simulink model "TSR_Scenario_002_cs"  (R2014b)
(part 2 of 39)

      mask help:
      | The VisuMatrixSign block provides a way to adapt the texture of the plates connected to an overhang, based on Resource IDs of the texture files.
      |
      | For more information, please click Help.
      settings: OpenFcn=open_system([gcb '/Actuator'],'mask')
      mask Help: eval('openHelp(733)')
      mask Display: image(imread('HighwaySpeedMatrix.png'))
  VISUMatrixSign_HighwayOverhang_21 : Subsystem  Tag=actuator/VisuMatrixSign  Priority=0  mask(PreScan Sink Block: VisuMatrixSign){UniqueID=1099, ResourceList={'1' 'InformationSign\MatrixSign_GreenArrow.png' '2' 'InformationSign\Empty.jpeg' '3' 'InformationSign\SEARCH_Logo.png' '4' 'InformationSign\z274-50_black_full.png' '5' 'InformationSign\z274-51_black_full.png' '6' 'InformationSign\z274-52_black_full.png' '7' 'InformationSign\z274-53_black_full.png' '8' 'InformationSign\z274-54_black_full.png' '9' 'InformationSign\z274-55_black_full.png' '10' 'InformationSign\z274-56_black_full.png' '11' 'InformationSign\z274-57_black_full.png' '12' 'InformationSign\z274-58_black_full.png' '13' 'InformationSign\z274-59_black_full.png' '14' 'InformationSign\z274-60_black_full.png' '15' 'InformationSign\z274-61_black_full.png' '16' 'InformationSign\z274-62_black_full.png' '17' 'InformationSign\z274-63_black_full.png' }, PivotName=}
      mask prompts: UniqueID "Parent Unique Identifier (auto-generated)"; ResourceList "Resource List (auto-generated)"; PivotName "Name of pivot (auto-generated)"
      mask help:
      | The VisuMatrixSign block provides a way to adapt the texture of the plates connected to an overhang, based on Resource IDs of the texture files.
      |
      | For more information, please click Help.
      settings: OpenFcn=open_system([gcb '/Actuator'],'mask')
      mask Help: eval('openHelp(733)')
      mask Display: image(imread('HighwaySpeedMatrix.png'))
  VISUMatrixSign_HighwayOverhang_22 : Subsystem  Tag=actuator/VisuMatrixSign  Priority=0  mask(PreScan Sink Block: VisuMatrixSign){UniqueID=1100, ResourceList={'1' 'InformationSign\MatrixSign_GreenArrow.png' '2' 'InformationSign\Empty.jpeg' '3' 'InformationSign\SEARCH_Logo.png' '4' 'InformationSign\z274-50_black_full.png' '5' 'InformationSign\z274-51_black_full.png' '6' 'InformationSign\z274-52_black_full.png' '7' 'InformationSign\z274-53_black_full.png' '8' 'InformationSign\z274-54_black_full.png' '9' 'InformationSign\z274-55_black_full.png' '10' 'InformationSign\z274-56_black_full.png' '11' 'InformationSign\z274-57_black_full.png' '12' 'InformationSign\z274-58_black_full.png' '13' 'InformationSign\z274-59_black_full.png' '14' 'InformationSign\z274-60_black_full.png' '15' 'InformationSign\z274-61_black_full.png' '16' 'InformationSign\z274-62_black_full.png' '17' 'InformationSign\z274-63_black_full.png' }, PivotName=}
      mask prompts: UniqueID "Parent Unique Identifier (auto-generated)"; ResourceList "Resource List (auto-generated)"; PivotName "Name of pivot (auto-generated)"
      mask help:
      | The VisuMatrixSign block provides a way to adapt the texture of the plates connected to an overhang, based on Resource IDs of the texture files.
      |
      | For more information, please click Help.
      settings: OpenFcn=open_system([gcb '/Actuator'],'mask')
      mask Help: eval('openHelp(733)')
      mask Display: image(imread('HighwaySpeedMatrix.png'))
  VISUMatrixSign_HighwayOverhang_23 : Subsystem  Tag=actuator/VisuMatrixSign  Priority=0  mask(PreScan Sink Block: VisuMatrixSign){UniqueID=1102, ResourceList={'1' 'InformationSign\MatrixSign_GreenArrow.png' '2' 'InformationSign\Empty.jpeg' '3' 'InformationSign\SEARCH_Logo.png' '4' 'InformationSign\z274-50_black_full.png' '5' 'InformationSign\z274-51_black_full.png' '6' 'InformationSign\z274-52_black_full.png' '7' 'InformationSign\z274-53_black_full.png' '8' 'InformationSign\z274-54_black_full.png' '9' 'InformationSign\z274-55_black_full.png' '10' 'InformationSign\z274-56_black_full.png' '11' 'InformationSign\z274-57_black_full.png' '12' 'InformationSign\z274-58_black_full.png' '13' 'InformationSign\z274-59_black_full.png' '14' 'InformationSign\z274-60_black_full.png' '15' 'InformationSign\z274-61_black_full.png' '16' 'InformationSign\z274-62_black_full.png' '17' 'InformationSign\z274-63_black_full.png' }, PivotName=}
      mask prompts: UniqueID "Parent Unique Identifier (auto-generated)"; ResourceList "Resource List (auto-generated)"; PivotName "Name of pivot (auto-generated)"
      mask help:
      | The VisuMatrixSign block provides a way to adapt the texture of the plates connected to an overhang, based on Resource IDs of the texture files.
      |
      | For more information, please click Help.
      settings: OpenFcn=open_system([gcb '/Actuator'],'mask')
      mask Help: eval('openHelp(733)')
      mask Display: image(imread('HighwaySpeedMatrix.png'))
  VISUMatrixSign_HighwayOverhang_24 : Subsystem  Tag=actuator/VisuMatrixSign  Priority=0  mask(PreScan Sink Block: VisuMatrixSign){UniqueID=1103, ResourceList={'1' 'InformationSign\MatrixSign_GreenArrow.png' '2' 'InformationSign\Empty.jpeg' '3' 'InformationSign\SEARCH_Logo.png' '4' 'InformationSign\z274-50_black_full.png' '5' 'InformationSign\z274-51_black_full.png' '6' 'InformationSign\z274-52_black_full.png' '7' 'InformationSign\z274-53_black_full.png' '8' 'InformationSign\z274-54_black_full.png' '9' 'InformationSign\z274-55_black_full.png' '10' 'InformationSign\z274-56_black_full.png' '11' 'InformationSign\z274-57_black_full.png' '12' 'InformationSign\z274-58_black_full.png' '13' 'InformationSign\z274-59_black_full.png' '14' 'InformationSign\z274-60_black_full.png' '15' 'InformationSign\z274-61_black_full.png' '16' 'InformationSign\z274-62_black_full.png' '17' 'InformationSign\z274-63_black_full.png' }, PivotName=}
      mask prompts: UniqueID "Parent Unique Identifier (auto-generated)"; ResourceList "Resource List (auto-generated)"; PivotName "Name of pivot (auto-generated)"
      mask help:
      | The VisuMatrixSign block provides a way to adapt the texture of the plates connected to an overhang, based on Resource IDs of the texture files.
      |
      | For more information, please click Help.
      settings: OpenFcn=open_system([gcb '/Actuator'],'mask')
      mask Help: eval('openHelp(733)')
      mask Display: image(imread('HighwaySpeedMatrix.png'))
  VISUMatrixSign_HighwayOverhang_25 : Subsystem  Tag=actuator/VisuMatrixSign  Priority=0  mask(PreScan Sink Block: VisuMatrixSign){UniqueID=1104, ResourceList={'1' 'InformationSign\MatrixSign_GreenArrow.png' '2' 'InformationSign\Empty.jpeg' '3' 'InformationSign\SEARCH_Logo.png' '4' 'InformationSign\z274-50_black_full.png' '5' 'InformationSign\z274-51_black_full.png' '6' 'InformationSign\z274-52_black_full.png' '7' 'InformationSign\z274-53_black_full.png' '8' 'InformationSign\z274-54_black_full.png' '9' 'InformationSign\z274-55_black_full.png' '10' 'InformationSign\z274-56_black_full.png' '11' 'InformationSign\z274-57_black_full.png' '12' 'InformationSign\z274-58_black_full.png' '13' 'InformationSign\z274-59_black_full.png' '14' 'InformationSign\z274-60_black_full.png' '15' 'InformationSign\z274-61_black_full.png' '16' 'InformationSign\z274-62_black_full.png' '17' 'InformationSign\z274-63_black_full.png' }, PivotName=}
      mask prompts: UniqueID "Parent Unique Identifier (auto-generated)"; ResourceList "Resource List (auto-generated)"; PivotName "Name of pivot (auto-generated)"
      mask help:
      | The VisuMatrixSign block provides a way to adapt the texture of the plates connected to an overhang, based on Resource IDs of the texture files.
      |
      | For more information, please click Help.
      settings: OpenFcn=open_system([gcb '/Actuator'],'mask')
      mask Help: eval('openHelp(733)')
      mask Display: image(imread('HighwaySpeedMatrix.png'))
  VISUMatrixSign_HighwayOverhang_26 : Subsystem  Tag=actuator/VisuMatrixSign  Priority=0  mask(PreScan Sink Block: VisuMatrixSign){UniqueID=1105, ResourceList={'1' 'InformationSign\MatrixSign_GreenArrow.png' '2' 'InformationSign\Empty.jpeg' '3' 'InformationSign\SEARCH_Logo.png' '4' 'InformationSign\z274-50_black_full.png' '5' 'InformationSign\z274-51_black_full.png' '6' 'InformationSign\z274-52_black_full.png' '7' 'InformationSign\z274-53_black_full.png' '8' 'InformationSign\z274-54_black_full.png' '9' 'InformationSign\z274-55_black_full.png' '10' 'InformationSign\z274-56_black_full.png' '11' 'InformationSign\z274-57_black_full.png' '12' 'InformationSign\z274-58_black_full.png' '13' 'InformationSign\z274-59_black_full.png' '14' 'InformationSign\z274-60_black_full.png' '15' 'InformationSign\z274-61_black_full.png' '16' 'InformationSign\z274-62_black_full.png' '17' 'InformationSign\z274-63_black_full.png' }, PivotName=}
      mask prompts: UniqueID "Parent Unique Identifier (auto-generated)"; ResourceList "Resource List (auto-generated)"; PivotName "Name of pivot (auto-generated)"
      mask help:
      | The VisuMatrixSign block provides a way to adapt the texture of the plates connected to an overhang, based on Resource IDs of the texture files.
      |
      | For more information, please click Help.
      settings: OpenFcn=open_system([gcb '/Actuator'],'mask')
      mask Help: eval('openHelp(733)')
      mask Display: image(imread('HighwaySpeedMatrix.png'))
  VISUMatrixSign_HighwayOverhang_27 : Subsystem  Tag=actuator/VisuMatrixSign  Priority=0  mask(PreScan Sink Block: VisuMatrixSign){UniqueID=1106, ResourceList={'1' 'InformationSign\MatrixSign_GreenArrow.png' '2' 'InformationSign\Empty.jpeg' '3' 'InformationSign\SEARCH_Logo.png' '4' 'InformationSign\z274-50_black_full.png' '5' 'InformationSign\z274-51_black_full.png' '6' 'InformationSign\z274-52_black_full.png' '7' 'InformationSign\z274-53_black_full.png' '8' 'InformationSign\z274-54_black_full.png' '9' 'InformationSign\z274-55_black_full.png' '10' 'InformationSign\z274-56_black_full.png' '11' 'InformationSign\z274-57_black_full.png' '12' 'InformationSign\z274-58_black_full.png' '13' 'InformationSign\z274-59_black_full.png' '14' 'InformationSign\z274-60_black_full.png' '15' 'InformationSign\z274-61_black_full.png' '16' 'InformationSign\z274-62_black_full.png' '17' 'InformationSign\z274-63_black_full.png' }, PivotName=}
      mask prompts: UniqueID "Parent Unique Identifier (auto-generated)"; ResourceList "Resource List (auto-generated)"; PivotName "Name of pivot (auto-generated)"
      mask help:
      | The VisuMatrixSign block provides a way to adapt the texture of the plates connected to an overhang, based on Resource IDs of the texture files.
      |
      | For more information, please click Help.
      settings: OpenFcn=open_system([gcb '/Actuator'],'mask')
      mask Help: eval('openHelp(733)')
      mask Display: image(imread('HighwaySpeedMatrix.png'))
  VISUMatrixSign_HighwayOverhang_28 : Subsystem  Tag=actuator/VisuMatrixSign  Priority=0  mask(PreScan Sink Block: VisuMatrixSign){UniqueID=1107, ResourceList={'1' 'InformationSign\MatrixSign_GreenArrow.png' '2' 'InformationSign\Empty.jpeg' '3' 'InformationSign\SEARCH_Logo.png' '4' 'InformationSign\z274-50_black_full.png' '5' 'InformationSign\z274-51_black_full.png' '6' 'InformationSign\z274-52_black_full.png' '7' 'InformationSign\z274-53_black_full.png' '8' 'InformationSign\z274-54_black_full.png' '9' 'InformationSign\z274-55_black_full.png' '10' 'InformationSign\z274-56_black_full.png' '11' 'InformationSign\z274-57_black_full.png' '12' 'InformationSign\z274-58_black_full.png' '13' 'InformationSign\z274-59_black_full.png' '14' 'InformationSign\z274-60_black_full.png' '15' 'InformationSign\z274-61_black_full.png' '16' 'InformationSign\z274-62_black_full.png' '17' 'InformationSign\z274-63_black_full.png' }, PivotName=}
      mask prompts: UniqueID "Parent Unique Identifier (auto-generated)"; ResourceList "Resource List (auto-generated)"; PivotName "Name of pivot (auto-generated)"
      mask help:
      | The VisuMatrixSign block provides a way to adapt the texture of the plates connected to an overhang, based on Resource IDs of the texture files.
      |
      | For more information, please click Help.
      settings: OpenFcn=open_system([gcb '/Actuator'],'mask')
      mask Help: eval('openHelp(733)')
      mask Display: image(imread('HighwaySpeedMatrix.png'))
  VISUMatrixSign_HighwayOverhang_3 : Subsystem  Tag=actuator/VisuMatrixSign  Priority=0  mask(PreScan Sink Block: VisuMatrixSign){UniqueID=440, ResourceList={'1' 'InformationSign\MatrixSign_GreenArrow.png' '2' 'InformationSign\Empty.jpeg' '3' 'InformationSign\SEARCH_Logo.png' '4' 'InformationSign\z274-50_black_full.png' '5' 'InformationSign\z274-51_black_full.png' '6' 'InformationSign\z274-52_black_full.png' '7' 'InformationSign\z274-53_black_full.png' '8' 'InformationSign\z274-54_black_full.png' '9' 'InformationSign\z274-55_black_full.png' '10' 'InformationSign\z274-56_black_full.png' '11' 'InformationSign\z274-57_black_full.png' '12' 'InformationSign\z274-58_black_full.png' '13' 'InformationSign\z274-59_black_full.png' '14' 'InformationSign\z274-60_black_full.png' '15' 'InformationSign\z274-61_black_full.png' '16' 'InformationSign\z274-62_black_full.png' '17' 'InformationSign\z274-63_black_full.png' }, PivotName=}
      mask prompts: UniqueID "Parent Unique Identifier (auto-generated)"; ResourceList "Resource List (auto-generated)"; PivotName "Name of pivot (auto-generated)"
      mask help:
      | The VisuMatrixSign block provides a way to adapt the texture of the plates connected to an overhang, based on Resource IDs of the texture files.
      |
      | For more information, please click Help.
      settings: OpenFcn=open_system([gcb '/Actuator'],'mask')
      mask Help: eval('openHelp(733)')
      mask Display: image(imread('HighwaySpeedMatrix.png'))
  VISUMatrixSign_HighwayOverhang_4 : Subsystem  Tag=actuator/VisuMatrixSign  Priority=0  mask(PreScan Sink Block: VisuMatrixSign){UniqueID=441, ResourceList={'1' 'InformationSign\MatrixSign_GreenArrow.png' '2' 'InformationSign\Empty.jpeg' '3' 'InformationSign\SEARCH_Logo.png' '4' 'InformationSign\z274-50_black_full.png' '5' 'InformationSign\z274-51_black_full.png' '6' 'InformationSign\z274-52_black_full.png' '7' 'InformationSign\z274-53_black_full.png' '8' 'InformationSign\z274-54_black_full.png' '9' 'InformationSign\z274-55_black_full.png' '10' 'InformationSign\z274-56_black_full.png' '11' 'InformationSign\z274-57_black_full.png' '12' 'InformationSign\z274-58_black_full.png' '13' 'InformationSign\z274-59_black_full.png' '14' 'InformationSign\z274-60_black_full.png' '15' 'InformationSign\z274-61_black_full.png' '16' 'InformationSign\z274-62_black_full.png' '17' 'InformationSign\z274-63_black_full.png' }, PivotName=}
      mask prompts: UniqueID "Parent Unique Identifier (auto-generated)"; ResourceList "Resource List (auto-generated)"; PivotName "Name of pivot (auto-generated)"
      mask help:
      | The VisuMatrixSign block provides a way to adapt the texture of the plates connected to an overhang, based on Resource IDs of the texture files.
      |
      | For more information, please click Help.
      settings: OpenFcn=open_system([gcb '/Actuator'],'mask')
      mask Help: eval('openHelp(733)')
      mask Display: image(imread('HighwaySpeedMatrix.png'))
  VISUMatrixSign_HighwayOverhang_5 : Subsystem  Tag=actuator/VisuMatrixSign  Priority=0  mask(PreScan Sink Block: VisuMatrixSign){UniqueID=843, ResourceList={'1' 'InformationSign\MatrixSign_GreenArrow.png' '2' 'InformationSign\Empty.jpeg' '3' 'InformationSign\SEARCH_Logo.png' '4' 'InformationSign\z274-50_black_full.png' '5' 'InformationSign\z274-51_black_full.png' '6' 'InformationSign\z274-52_black_full.png' '7' 'InformationSign\z274-53_black_full.png' '8' 'InformationSign\z274-54_black_full.png' '9' 'InformationSign\z274-55_black_full.png' '10' 'InformationSign\z274-56_black_full.png' '11' 'InformationSign\z274-57_black_full.png' '12' 'InformationSign\z274-58_black_full.png' '13' 'InformationSign\z274-59_black_full.png' '14' 'InformationSign\z274-60_black_full.png' '15' 'InformationSign\z274-61_black_full.png' '16' 'InformationSign\z274-62_black_full.png' '17' 'InformationSign\z274-63_black_full.png' }, PivotName=}
      mask prompts: UniqueID "Parent Unique Identifier (auto-generated)"; ResourceList "Resource List (auto-generated)"; PivotName "Name of pivot (auto-generated)"
      mask help:
      | The VisuMatrixSign block provides a way to adapt the texture of the plates connected to an overhang, based on Resource IDs of the texture files.
      |
      | For more information, please click Help.
      settings: OpenFcn=open_system([gcb '/Actuator'],'mask')
      mask Help: eval('openHelp(733)')
      mask Display: image(imread('HighwaySpeedMatrix.png'))
  VISUMatrixSign_HighwayOverhang_6 : Subsystem  Tag=actuator/VisuMatrixSign  Priority=0  mask(PreScan Sink Block: VisuMatrixSign){UniqueID=846, ResourceList={'1' 'InformationSign\MatrixSign_GreenArrow.png' '2' 'InformationSign\Empty.jpeg' '3' 'InformationSign\SEARCH_Logo.png' '4' 'InformationSign\z274-50_black_full.png' '5' 'InformationSign\z274-51_black_full.png' '6' 'InformationSign\z274-52_black_full.png' '7' 'InformationSign\z274-53_black_full.png' '8' 'InformationSign\z274-54_black_full.png' '9' 'InformationSign\z274-55_black_full.png' '10' 'InformationSign\z274-56_black_full.png' '11' 'InformationSign\z274-57_black_full.png' '12' 'InformationSign\z274-58_black_full.png' '13' 'InformationSign\z274-59_black_full.png' '14' 'InformationSign\z274-60_black_full.png' '15' 'InformationSign\z274-61_black_full.png' '16' 'InformationSign\z274-62_black_full.png' '17' 'InformationSign\z274-63_black_full.png' }, PivotName=}
      mask prompts: UniqueID "Parent Unique Identifier (auto-generated)"; ResourceList "Resource List (auto-generated)"; PivotName "Name of pivot (auto-generated)"
      mask help:
      | The VisuMatrixSign block provides a way to adapt the texture of the plates connected to an overhang, based on Resource IDs of the texture files.
      |
      | For more information, please click Help.
      settings: OpenFcn=open_system([gcb '/Actuator'],'mask')
      mask Help: eval('openHelp(733)')
      mask Display: image(imread('HighwaySpeedMatrix.png'))
  VISUMatrixSign_HighwayOverhang_7 : Subsystem  Tag=actuator/VisuMatrixSign  Priority=0  mask(PreScan Sink Block: VisuMatrixSign){UniqueID=867, ResourceList={'1' 'InformationSign\MatrixSign_GreenArrow.png' '2' 'InformationSign\Empty.jpeg' '3' 'InformationSign\SEARCH_Logo.png' '4' 'InformationSign\z274-50_black_full.png' '5' 'InformationSign\z274-51_black_full.png' '6' 'InformationSign\z274-52_black_full.png' '7' 'InformationSign\z274-53_black_full.png' '8' 'InformationSign\z274-54_black_full.png' '9' 'InformationSign\z274-55_black_full.png' '10' 'InformationSign\z274-56_black_full.png' '11' 'InformationSign\z274-57_black_full.png' '12' 'InformationSign\z274-58_black_full.png' '13' 'InformationSign\z274-59_black_full.png' '14' 'InformationSign\z274-60_black_full.png' '15' 'InformationSign\z274-61_black_full.png' '16' 'InformationSign\z274-62_black_full.png' '17' 'InformationSign\z274-63_black_full.png' }, PivotName=}
      mask prompts: UniqueID "Parent Unique Identifier (auto-generated)"; ResourceList "Resource List (auto-generated)"; PivotName "Name of pivot (auto-generated)"
      mask help:
      | The VisuMatrixSign block provides a way to adapt the texture of the plates connected to an overhang, based on Resource IDs of the texture files.
      |
      | For more information, please click Help.
      settings: OpenFcn=open_system([gcb '/Actuator'],'mask')
      mask Help: eval('openHelp(733)')
      mask Display: image(imread('HighwaySpeedMatrix.png'))
  VISUMatrixSign_HighwayOverhang_8 : Subsystem  Tag=actuator/VisuMatrixSign  Priority=0  mask(PreScan Sink Block: VisuMatrixSign){UniqueID=870, ResourceList={'1' 'InformationSign\MatrixSign_GreenArrow.png' '2' 'InformationSign\Empty.jpeg' '3' 'InformationSign\SEARCH_Logo.png' '4' 'InformationSign\z274-50_black_full.png' '5' 'InformationSign\z274-51_black_full.png' '6' 'InformationSign\z274-52_black_full.png' '7' 'InformationSign\z274-53_black_full.png' '8' 'InformationSign\z274-54_black_full.png' '9' 'InformationSign\z274-55_black_full.png' '10' 'InformationSign\z274-56_black_full.png' '11' 'InformationSign\z274-57_black_full.png' '12' 'InformationSign\z274-58_black_full.png' '13' 'InformationSign\z274-59_black_full.png' '14' 'InformationSign\z274-60_black_full.png' '15' 'InformationSign\z274-61_black_full.png' '16' 'InformationSign\z274-62_black_full.png' '17' 'InformationSign\z274-63_black_full.png' }, PivotName=}
      mask prompts: UniqueID "Parent Unique Identifier (auto-generated)"; ResourceList "Resource List (auto-generated)"; PivotName "Name of pivot (auto-generated)"
      mask help:
      | The VisuMatrixSign block provides a way to adapt the texture of the plates connected to an overhang, based on Resource IDs of the texture files.
      |
      | For more information, please click Help.
      settings: OpenFcn=open_system([gcb '/Actuator'],'mask')
      mask Help: eval('openHelp(733)')
      mask Display: image(imread('HighwaySpeedMatrix.png'))
  VISUMatrixSign_HighwayOverhang_9 : Subsystem  Tag=actuator/VisuMatrixSign  Priority=0  mask(PreScan Sink Block: VisuMatrixSign){UniqueID=875, ResourceList={'1' 'InformationSign\MatrixSign_GreenArrow.png' '2' 'InformationSign\Empty.jpeg' '3' 'InformationSign\SEARCH_Logo.png' '4' 'InformationSign\z274-50_black_full.png' '5' 'InformationSign\z274-51_black_full.png' '6' 'InformationSign\z274-52_black_full.png' '7' 'InformationSign\z274-53_black_full.png' '8' 'InformationSign\z274-54_black_full.png' '9' 'InformationSign\z274-55_black_full.png' '10' 'InformationSign\z274-56_black_full.png' '11' 'InformationSign\z274-57_black_full.png' '12' 'InformationSign\z274-58_black_full.png' '13' 'InformationSign\z274-59_black_full.png' '14' 'InformationSign\z274-60_black_full.png' '15' 'InformationSign\z274-61_black_full.png' '16' 'InformationSign\z274-62_black_full.png' '17' 'InformationSign\z274-63_black_full.png' }, PivotName=}
      mask prompts: UniqueID "Parent Unique Identifier (auto-generated)"; ResourceList "Resource List (auto-generated)"; PivotName "Name of pivot (auto-generated)"
      mask help:
      | The VisuMatrixSign block provides a way to adapt the texture of the plates connected to an overhang, based on Resource IDs of the texture files.
      |
      | For more information, please click Help.
      settings: OpenFcn=open_system([gcb '/Actuator'],'mask')
      mask Help: eval('openHelp(733)')
      mask Display: image(imread('HighwaySpeedMatrix.png'))
  WheelL0_Audi_A8_1 : Subsystem  Tag=Actuator  Priority=0  LoadFcn=load('PrescanPoseData');load('PrescanXYZData');load('PreScanRPYData')
      mask help:
      | The VisuJoint block provides a way to adapt the location and orientation of a part of an object.
      |
      | For more information, please click Help.
      settings: OpenFcn=open_system([gcb '/Actuator'],'mask')
      mask Display: image(imread('Joint.png'))
  WheelL0_BMW_X5_2 : Subsystem  Tag=Actuator  Priority=0  LoadFcn=load('PrescanPoseData');load('PrescanXYZData');load('PreScanRPYData')
      mask help:
      | The VisuJoint block provides a way to adapt the location and orientation of a part of an object.
      |
      | For more information, please click Help.
      settings: OpenFcn=open_system([gcb '/Actuator'],'mask')
      mask Display: image(imread('Joint.png'))
  WheelL0_Citroen_C3_1 : Subsystem  Tag=Actuator  Priority=0  LoadFcn=load('PrescanPoseData');load('PrescanXYZData');load('PreScanRPYData')
      mask help:
      | The VisuJoint block provides a way to adapt the location and orientation of a part of an object.
      |
      | For more information, please click Help.
      settings: OpenFcn=open_system([gcb '/Actuator'],'mask')
      mask Display: image(imread('Joint.png'))
  WheelL0_Fiat_Bravo_1 : Subsystem  Tag=Actuator  Priority=0  LoadFcn=load('PrescanPoseData');load('PrescanXYZData');load('PreScanRPYData')
      mask help:
      | The VisuJoint block provides a way to adapt the location and orientation of a part of an object.
      |
      | For more information, please click Help.
      settings: OpenFcn=open_system([gcb '/Actuator'],'mask')
      mask Display: image(imread('Joint.png'))
  WheelL0_Nissan_Cabstar_1 : Subsystem  Tag=Actuator  Priority=0  LoadFcn=load('PrescanPoseData');load('PrescanXYZData');load('PreScanRPYData')
      mask help:
      | The VisuJoint block provides a way to adapt the location and orientation of a part of an object.
      |
      | For more information, please click Help.
      settings: OpenFcn=open_system([gcb '/Actuator'],'mask')
      mask Display: image(imread('Joint.png'))
  WheelL1_Audi_A8_1 : Subsystem  Tag=Actuator  Priority=0  LoadFcn=load('PrescanPoseData');load('PrescanXYZData');load('PreScanRPYData')
      mask help:
      | The VisuJoint block provides a way to adapt the location and orientation of a part of an object.
      |
      | For more information, please click Help.
      settings: OpenFcn=open_system([gcb '/Actuator'],'mask')
      mask Display: image(imread('Joint.png'))
  WheelL1_BMW_X5_2 : Subsystem  Tag=Actuator  Priority=0  LoadFcn=load('PrescanPoseData');load('PrescanXYZData');load('PreScanRPYData')
      mask help:
      | The VisuJoint block provides a way to adapt the location and orientation of a part of an object.
      |
      | For more information, please click Help.
      settings: OpenFcn=open_system([gcb '/Actuator'],'mask')
      mask Display: image(imread('Joint.png'))
  WheelL1_Citroen_C3_1 : Subsystem  Tag=Actuator  Priority=0  LoadFcn=load('PrescanPoseData');load('PrescanXYZData');load('PreScanRPYData')
      mask help:
      | The VisuJoint block provides a way to adapt the location and orientation of a part of an object.
      |
      | For more information, please click Help.
      settings: OpenFcn=open_system([gcb '/Actuator'],'mask')
      mask Display: image(imread('Joint.png'))
  WheelL1_Fiat_Bravo_1 : Subsystem  Tag=Actuator  Priority=0  LoadFcn=load('PrescanPoseData');load('PrescanXYZData');load('PreScanRPYData')
      mask help:
      | The VisuJoint block provides a way to adapt the location and orientation of a part of an object.
      |
      | For more information, please click Help.
      settings: OpenFcn=open_system([gcb '/Actuator'],'mask')
      mask Display: image(imread('Joint.png'))
  WheelL1_Nissan_Cabstar_1 : Subsystem  Tag=Actuator  Priority=0  LoadFcn=load('PrescanPoseData');load('PrescanXYZData');load('PreScanRPYData')
      mask help:
      | The VisuJoint block provides a way to adapt the location and orientation of a part of an object.
      |
      | For more information, please click Help.
      settings: OpenFcn=open_system([gcb '/Actuator'],'mask')
      mask Display: image(imread('Joint.png'))
  WheelR0_Audi_A8_1 : Subsystem  Tag=Actuator  Priority=0  LoadFcn=load('PrescanPoseData');load('PrescanXYZData');load('PreScanRPYData')
      mask help:
      | The VisuJoint block provides a way to adapt the location and orientation of a part of an object.
      |
      | For more information, please click Help.
      settings: OpenFcn=open_system([gcb '/Actuator'],'mask')
      mask Display: image(imread('Joint.png'))
  WheelR0_BMW_X5_2 : Subsystem  Tag=Actuator  Priority=0  LoadFcn=load('PrescanPoseData');load('PrescanXYZData');load('PreScanRPYData')
      mask help:
      | The VisuJoint block provides a way to adapt the location and orientation of a part of an object.
      |
      | For more information, please click Help.
      settings: OpenFcn=open_system([gcb '/Actuator'],'mask')
      mask Display: image(imread('Joint.png'))
  WheelR0_Citroen_C3_1 : Subsystem  Tag=Actuator  Priority=0  LoadFcn=load('PrescanPoseData');load('PrescanXYZData');load('PreScanRPYData')
      mask help:
      | The VisuJoint block provides a way to adapt the location and orientation of a part of an object.
      |
      | For more information, please click Help.
      settings: OpenFcn=open_system([gcb '/Actuator'],'mask')
      mask Display: image(imread('Joint.png'))
  WheelR0_Fiat_Bravo_1 : Subsystem  Tag=Actuator  Priority=0  LoadFcn=load('PrescanPoseData');load('PrescanXYZData');load('PreScanRPYData')
      mask help:
      | The VisuJoint block provides a way to adapt the location and orientation of a part of an object.
      |
      | For more information, please click Help.
      settings: OpenFcn=open_system([gcb '/Actuator'],'mask')
      mask Display: image(imread('Joint.png'))
  WheelR0_Nissan_Cabstar_1 : Subsystem  Tag=Actuator  Priority=0  LoadFcn=load('PrescanPoseData');load('PrescanXYZData');load('PreScanRPYData')
      mask help:
      | The VisuJoint block provides a way to adapt the location and orientation of a part of an object.
      |
      | For more information, please click Help.
      settings: OpenFcn=open_system([gcb '/Actuator'],'mask')
      mask Display: image(imread('Joint.png'))
  WheelR1_Audi_A8_1 : Subsystem  Tag=Actuator  Priority=0  LoadFcn=load('PrescanPoseData');load('PrescanXYZData');load('PreScanRPYData')
      mask help:
      | The VisuJoint block provides a way to adapt the location and orientation of a part of an object.
      |
      | For more information, please click Help.
      settings: OpenFcn=open_system([gcb '/Actuator'],'mask')
      mask Display: image(imread('Joint.png'))
  WheelR1_BMW_X5_2 : Subsystem  Tag=Actuator  Priority=0  LoadFcn=load('PrescanPoseData');load('PrescanXYZData');load('PreScanRPYData')
      mask help:
      | The VisuJoint block provides a way to adapt the location and orientation of a part of an object.
      |
      | For more information, please click Help.
      settings: OpenFcn=open_system([gcb '/Actuator'],'mask')
      mask Display: image(imread('Joint.png'))
  WheelR1_Citroen_C3_1 : Subsystem  Tag=Actuator  Priority=0  LoadFcn=load('PrescanPoseData');load('PrescanXYZData');load('PreScanRPYData')
      mask help:
      | The VisuJoint block provides a way to adapt the location and orientation of a part of an object.
      |
      | For more information, please click Help.
      settings: OpenFcn=open_system([gcb '/Actuator'],'mask')
      mask Display: image(imread('Joint.png'))
  WheelR1_Fiat_Bravo_1 : Subsystem  Tag=Actuator  Priority=0  LoadFcn=load('PrescanPoseData');load('PrescanXYZData');load('PreScanRPYData')
      mask help:
      | The VisuJoint block provides a way to adapt the location and orientation of a part of an object.
      |
      | For more information, please click Help.
      settings: OpenFcn=open_system([gcb '/Actuator'],'mask')
      mask Display: image(imread('Joint.png'))
  WheelR1_Nissan_Cabstar_1 : Subsystem  Tag=Actuator  Priority=0  LoadFcn=load('PrescanPoseData');load('PrescanXYZData');load('PreScanRPYData')
      mask help:
      | The VisuJoint block provides a way to adapt the location and orientation of a part of an object.
      |
      | For more information, please click Help.
      settings: OpenFcn=open_system([gcb '/Actuator'],'mask')
      mask Display: image(imread('Joint.png'))
  wires:
  Audi_A8_1/1(STATE_Audi_A8_1_bus) -> STATE_Audi_A8_1_bus/1(STATE_Audi_A8_1_bus)
  SELF_Audi_A8_1/1(SELF_Audi_A8_1) -> Audi_A8_1/1(SELF_Audi_A8_1)
  CameraSensor_1/1(CameraSensor_1) -> Audi_A8_1/2(CameraSensor_1)
  Audi_A8_1/2(WheelL0_Audi_A8_1) -> WheelL0_Audi_A8_1/1(WheelL0_Audi_A8_1)
  Audi_A8_1/3(WheelL1_Audi_A8_1) -> WheelL1_Audi_A8_1/1(WheelL1_Audi_A8_1)
  Audi_A8_1/4(WheelR0_Audi_A8_1) -> WheelR0_Audi_A8_1/1(WheelR0_Audi_A8_1)
  Audi_A8_1/5(WheelR1_Audi_A8_1) -> WheelR1_Audi_A8_1/1(WheelR1_Audi_A8_1)
  Audi_A8_1/6(SteeringWheel_pivot_Audi_A8_1) -> SteeringWheel_pivot_Audi_A8_1/1(SteeringWheel_pivot_Audi_A8_1)
  Audi_A8_1/7(SteeringColumn_pivot_Audi_A8_1) -> SteeringColumn_pivot_Audi_A8_1/1(SteeringColumn_pivot_Audi_A8_1)
  Audi_A8_1/8(Audi_A8_1_Brake_light_left) -> Audi_A8_1_Brake_light_left/1(Audi_A8_1_Brake_light_left)
  Audi_A8_1/9(Audi_A8_1_Brake_light_right) -> Audi_A8_1_Brake_light_right/1(Audi_A8_1_Brake_light_right)
  Audi_A8_1/10(Audi_A8_1_Indicator_front_left) -> Audi_A8_1_Indicator_front_left/1(Audi_A8_1_Indicator_front_left)
  Audi_A8_1/11(Audi_A8_1_Indicator_rear_left) -> Audi_A8_1_Indicator_rear_left/1(Audi_A8_1_Indicator_rear_left)
  Audi_A8_1/12(Audi_A8_1_Indicator_front_right) -> Audi_A8_1_Indicator_front_right/1(Audi_A8_1_Indicator_front_right)
  Audi_A8_1/13(Audi_A8_1_Indicator_rear_right) -> Audi_A8_1_Indicator_rear_right/1(Audi_A8_1_Indicator_rear_right)
  Sphere_1/1(STATE_Sphere_1_bus) -> STATE_Sphere_1_bus/1(STATE_Sphere_1_bus)
  SELF_Sphere_1/1(SELF_Sphere_1) -> Sphere_1/1(SELF_Sphere_1)
  Nissan_Cabstar_1/1(STATE_Nissan_Cabstar_1_bus) -> STATE_Nissan_Cabstar_1_bus/1(STATE_Nissan_Cabstar_1_bus)
  SELF_Nissan_Cabstar_1/1(SELF_Nissan_Cabstar_1) -> Nissan_Cabstar_1/1(SELF_Nissan_Cabstar_1)
  Nissan_Cabstar_1/2(WheelL0_Nissan_Cabstar_1) -> WheelL0_Nissan_Cabstar_1/1(WheelL0_Nissan_Cabstar_1)
  Nissan_Cabstar_1/3(WheelL1_Nissan_Cabstar_1) -> WheelL1_Nissan_Cabstar_1/1(WheelL1_Nissan_Cabstar_1)
  Nissan_Cabstar_1/4(WheelR0_Nissan_Cabstar_1) -> WheelR0_Nissan_Cabstar_1/1(WheelR0_Nissan_Cabstar_1)
  Nissan_Cabstar_1/5(WheelR1_Nissan_Cabstar_1) -> WheelR1_Nissan_Cabstar_1/1(WheelR1_Nissan_Cabstar_1)
  Nissan_Cabstar_1/6(SteeringWheel_pivot_Nissan_Cabstar_1) -> SteeringWheel_pivot_Nissan_Cabstar_1/1(SteeringWheel_pivot_Nissan_Cabstar_1)
  Nissan_Cabstar_1/7(SteeringColumn_pivot_Nissan_Cabstar_1) -> SteeringColumn_pivot_Nissan_Cabstar_1/1(SteeringColumn_pivot_Nissan_Cabstar_1)
  Nissan_Cabstar_1/8(Nissan_Cabstar_1_Brake_light_left) -> Nissan_Cabstar_1_Brake_light_left/1(Nissan_Cabstar_1_Brake_light_left)
  Nissan_Cabstar_1/9(Nissan_Cabstar_1_Brake_light_right) -> Nissan_Cabstar_1_Brake_light_right/1(Nissan_Cabstar_1_Brake_light_right)
  Nissan_Cabstar_1/10(Nissan_Cabstar_1_Indicator_front_left) -> Nissan_Cabstar_1_Indicator_front_left/1(Nissan_Cabstar_1_Indicator_front_left)
  Nissan_Cabstar_1/11(Nissan_Cabstar_1_Indicator_side_left) -> Nissan_Cabstar_1_Indicator_side_left/1(Nissan_Cabstar_1_Indicator_side_left)
  Nissan_Cabstar_1/12(Nissan_Cabstar_1_Indicator_rear_left) -> Nissan_Cabstar_1_Indicator_rear_left/1(Nissan_Cabstar_1_Indicator_rear_left)
  Nissan_Cabstar_1/13(Nissan_Cabstar_1_Indicator_front_right) -> Nissan_Cabstar_1_Indicator_front_right/1(Nissan_Cabstar_1_Indicator_front_right)
  Nissan_Cabstar_1/14(Nissan_Cabstar_1_Indicator_side_right) -> Nissan_Cabstar_1_Indicator_side_right/1(Nissan_Cabstar_1_Indicator_side_right)
  Nissan_Cabstar_1/15(Nissan_Cabstar_1_Indicator_rear_right) -> Nissan_Cabstar_1_Indicator_rear_right/1(Nissan_Cabstar_1_Indicator_rear_right)
  Actros_2541_1/1(STATE_Actros_2541_1_bus) -> STATE_Actros_2541_1_bus/1(STATE_Actros_2541_1_bus)
  SELF_Actros_2541_1/1(SELF_Actros_2541_1) -> Actros_2541_1/1(SELF_Actros_2541_1)
  Actros_2541_1/2(SteeringWheel_pivot_Actros_2541_1) -> SteeringWheel_pivot_Actros_2541_1/1(SteeringWheel_pivot_Actros_2541_1)
  Actros_2541_1/3(SteeringColumn_pivot_Actros_2541_1) -> SteeringColumn_pivot_Actros_2541_1/1(SteeringColumn_pivot_Actros_2541_1)
  Actros_2541_1/4(Actros_2541_1_Brake_light_left) -> Actros_2541_1_Brake_light_left/1(Actros_2541_1_Brake_light_left)
  Actros_2541_1/5(Actros_2541_1_Brake_light_right) -> Actros_2541_1_Brake_light_right/1(Actros_2541_1_Brake_light_right)
  Actros_2541_1/6(Actros_2541_1_Indicator_front_left) -> Actros_2541_1_Indicator_front_left/1(Actros_2541_1_Indicator_front_left)
  Actros_2541_1/7(Actros_2541_1_Indicator_side_left_1) -> Actros_2541_1_Indicator_side_left_1/1(Actros_2541_1_Indicator_side_left_1)
  Actros_2541_1/8(Actros_2541_1_Indicator_side_left_2) -> Actros_2541_1_Indicator_side_left_2/1(Actros_2541_1_Indicator_side_left_2)
  Actros_2541_1/9(Actros_2541_1_Indicator_side_left_3) -> Actros_2541_1_Indicator_side_left_3/1(Actros_2541_1_Indicator_side_left_3)
  Actros_2541_1/10(Actros_2541_1_Indicator_rear_left) -> Actros_2541_1_Indicator_rear_left/1(Actros_2541_1_Indicator_rear_left)
  Actros_2541_1/11(Actros_2541_1_Indicator_front_right) -> Actros_2541_1_Indicator_front_right/1(Actros_2541_1_Indicator_front_right)
  Actros_2541_1/12(Actros_2541_1_Indicator_side_right_1) -> Actros_2541_1_Indicator_side_right_1/1(Actros_2541_1_Indicator_side_right_1)
  Actros_2541_1/13(Actros_2541_1_Indicator_side_right_2) -> Actros_2541_1_Indicator_side_right_2/1(Actros_2541_1_Indicator_side_right_2)
  Actros_2541_1/14(Actros_2541_1_Indicator_side_right_3) -> Actros_2541_1_Indicator_side_right_3/1(Actros_2541_1_Indicator_side_right_3)
  Actros_2541_1/15(Actros_2541_1_Indicator_rear_right) -> Actros_2541_1_Indicator_rear_right/1(Actros_2541_1_Indicator_rear_right)
  Actros_1860_1/1(STATE_Actros_1860_1_bus) -> STATE_Actros_1860_1_bus/1(STATE_Actros_1860_1_bus)
  SELF_Actros_1860_1/1(SELF_Actros_1860_1) -> Actros_1860_1/1(SELF_Actros_1860_1)
  Actros_1860_1/2(SteeringWheel_pivot_Actros_1860_1) -> SteeringWheel_pivot_Actros_1860_1/1(SteeringWheel_pivot_Actros_1860_1)
  Actros_1860_1/3(SteeringColumn_pivot_Actros_1860_1) -> SteeringColumn_pivot_Actros_1860_1/1(SteeringColumn_pivot_Actros_1860_1)
  Actros_1860_1/4(Actros_1860_1_Brake_light_left) -> Actros_1860_1_Brake_light_left/1(Actros_1860_1_Brake_light_left)
  Actros_1860_1/5(Actros_1860_1_Brake_light_right) -> Actros_1860_1_Brake_light_right/1(Actros_1860_1_Brake_light_right)
  Actros_1860_1/6(Actros_1860_1_Indicator_front_left) -> Actros_1860_1_Indicator_front_left/1(Actros_1860_1_Indicator_front_left)
  Actros_1860_1/7(Actros_1860_1_Indicator_side_left) -> Actros_1860_1_Indicator_side_left/1(Actros_1860_1_Indicator_side_left)
  Actros_1860_1/8(Actros_1860_1_Indicator_side_left_2) -> Actros_1860_1_Indicator_side_left_2/1(Actros_1860_1_Indicator_side_left_2)
  Actros_1860_1/9(Actros_1860_1_Indicator_side_left_3) -> Actros_1860_1_Indicator_side_left_3/1(Actros_1860_1_Indicator_side_left_3)
  Actros_1860_1/10(Actros_1860_1_Indicator_rear_left) -> Actros_1860_1_Indicator_rear_left/1(Actros_1860_1_Indicator_rear_left)
  Actros_1860_1/11(Actros_1860_1_Indicator_front_right) -> Actros_1860_1_Indicator_front_right/1(Actros_1860_1_Indicator_front_right)
  Actros_1860_1/12(Actros_1860_1_Indicator_side_right) -> Actros_1860_1_Indicator_side_right/1(Actros_1860_1_Indicator_side_right)
  Actros_1860_1/13(Actros_1860_1_Indicator_side_right_2) -> Actros_1860_1_Indicator_side_right_2/1(Actros_1860_1_Indicator_side_right_2)
  Actros_1860_1/14(Actros_1860_1_Indicator_side_right_3) -> Actros_1860_1_Indicator_side_right_3/1(Actros_1860_1_Indicator_side_right_3)
  Actros_1860_1/15(Actros_1860_1_Indicator_rear_right) -> Actros_1860_1_Indicator_rear_right/1(Actros_1860_1_Indicator_rear_right)
  BMW_X5_2/1(STATE_BMW_X5_2_bus) -> STATE_BMW_X5_2_bus/1(STATE_BMW_X5_2_bus)
  SELF_BMW_X5_2/1(SELF_BMW_X5_2) -> BMW_X5_2/1(SELF_BMW_X5_2)
  BMW_X5_2/2(WheelL0_BMW_X5_2) -> WheelL0_BMW_X5_2/1(WheelL0_BMW_X5_2)
  BMW_X5_2/3(WheelR0_BMW_X5_2) -> WheelR0_BMW_X5_2/1(WheelR0_BMW_X5_2)
  BMW_X5_2/4(WheelR1_BMW_X5_2) -> WheelR1_BMW_X5_2/1(WheelR1_BMW_X5_2)
  BMW_X5_2/5(WheelL1_BMW_X5_2) -> WheelL1_BMW_X5_2/1(WheelL1_BMW_X5_2)
  BMW_X5_2/6(SteeringWheel_pivot_BMW_X5_2) -> SteeringWheel_pivot_BMW_X5_2/1(SteeringWheel_pivot_BMW_X5_2)
  BMW_X5_2/7(SteeringColumn_pivot_BMW_X5_2) -> SteeringColumn_pivot_BMW_X5_2/1(SteeringColumn_pivot_BMW_X5_2)
  BMW_X5_2/8(BMW_X5_2_Brake_light_left) -> BMW_X5_2_Brake_light_left/1(BMW_X5_2_Brake_light_left)
  BMW_X5_2/9(BMW_X5_2_Brake_light_right) -> BMW_X5_2_Brake_light_right/1(BMW_X5_2_Brake_light_right)
  BMW_X5_2/10(BMW_X5_2_Indicator_front_left) -> BMW_X5_2_Indicator_front_left/1(BMW_X5_2_Indicator_front_left)
  BMW_X5_2/11(BMW_X5_2_Indicator_side_left) -> BMW_X5_2_Indicator_side_left/1(BMW_X5_2_Indicator_side_left)
  BMW_X5_2/12(BMW_X5_2_Indicator_rear_left) -> BMW_X5_2_Indicator_rear_left/1(BMW_X5_2_Indicator_rear_left)
  BMW_X5_2/13(BMW_X5_2_Indicator_front_right) -> BMW_X5_2_Indicator_front_right/1(BMW_X5_2_Indicator_front_right)
  BMW_X5_2/14(BMW_X5_2_Indicator_side_right) -> BMW_X5_2_Indicator_side_right/1(BMW_X5_2_Indicator_side_right)
  BMW_X5_2/15(BMW_X5_2_Indicator_rear_right) -> BMW_X5_2_Indicator_rear_right/1(BMW_X5_2_Indicator_rear_right)
  Citroen_C3_1/1(STATE_Citroen_C3_1_bus) -> STATE_Citroen_C3_1_bus/1(STATE_Citroen_C3_1_bus)
  SELF_Citroen_C3_1/1(SELF_Citroen_C3_1) -> Citroen_C3_1/1(SELF_Citroen_C3_1)
  Citroen_C3_1/2(WheelL0_Citroen_C3_1) -> WheelL0_Citroen_C3_1/1(WheelL0_Citroen_C3_1)
  Citroen_C3_1/3(WheelL1_Citroen_C3_1) -> WheelL1_Citroen_C3_1/1(WheelL1_Citroen_C3_1)
  Citroen_C3_1/4(WheelR0_Citroen_C3_1) -> WheelR0_Citroen_C3_1/1(WheelR0_Citroen_C3_1)
  Citroen_C3_1/5(WheelR1_Citroen_C3_1) -> WheelR1_Citroen_C3_1/1(WheelR1_Citroen_C3_1)
  Citroen_C3_1/6(SteeringWheel_Pivot_Citroen_C3_1) -> SteeringWheel_Pivot_Citroen_C3_1/1(SteeringWheel_Pivot_Citroen_C3_1)
  Citroen_C3_1/7(SteeringColumn_Pivot_Citroen_C3_1) -> SteeringColumn_Pivot_Citroen_C3_1/1(SteeringColumn_Pivot_Citroen_C3_1)
  Citroen_C3_1/8(Citroen_C3_1_Brake_light_left) -> Citroen_C3_1_Brake_light_left/1(Citroen_C3_1_Brake_light_left)
  Citroen_C3_1/9(Citroen_C3_1_Brake_light_right) -> Citroen_C3_1_Brake_light_right/1(Citroen_C3_1_Brake_light_right)
  Citroen_C3_1/10(Citroen_C3_1_Indicator_front_left) -> Citroen_C3_1_Indicator_front_left/1(Citroen_C3_1_Indicator_front_left)
  Citroen_C3_1/11(Citroen_C3_1_Indicator_side_left) -> Citroen_C3_1_Indicator_side_left/1(Citroen_C3_1_Indicator_side_left)
  Citroen_C3_1/12(Citroen_C3_1_Indicator_rear_left) -> Citroen_C3_1_Indicator_rear_left/1(Citroen_C3_1_Indicator_rear_left)
  Citroen_C3_1/13(Citroen_C3_1_Indicator_front_right) -> Citroen_C3_1_Indicator_front_right/1(Citroen_C3_1_Indicator_front_right)
  Citroen_C3_1/14(Citroen_C3_1_Indicator_side_right) -> Citroen_C3_1_Indicator_side_right/1(Citroen_C3_1_Indicator_side_right)
  Citroen_C3_1/15(Citroen_C3_1_Indicator_rear_right) -> Citroen_C3_1_Indicator_rear_right/1(Citroen_C3_1_Indicator_rear_right)
  Fiat_Bravo_1/1(STATE_Fiat_Bravo_1_bus) -> STATE_Fiat_Bravo_1_bus/1(STATE_Fiat_Bravo_1_bus)
  SELF_Fiat_Bravo_1/1(SELF_Fiat_Bravo_1) -> Fiat_Bravo_1/1(SELF_Fiat_Bravo_1)
  Fiat_Bravo_1/2(WheelL0_Fiat_Bravo_1) -> WheelL0_Fiat_Bravo_1/1(WheelL0_Fiat_Bravo_1)
  Fiat_Bravo_1/3(WheelL1_Fiat_Bravo_1) -> WheelL1_Fiat_Bravo_1/1(WheelL1_Fiat_Bravo_1)
  Fiat_Bravo_1/4(WheelR0_Fiat_Bravo_1) -> WheelR0_Fiat_Bravo_1/1(WheelR0_Fiat_Bravo_1)
  Fiat_Bravo_1/5(WheelR1_Fiat_Bravo_1) -> WheelR1_Fiat_Bravo_1/1(WheelR1_Fiat_Bravo_1)
  Fiat_Bravo_1/6(SteeringWheel_pivot_Fiat_Bravo_1) -> SteeringWheel_pivot_Fiat_Bravo_1/1(SteeringWheel_pivot_Fiat_Bravo_1)
  Fiat_Bravo_1/7(SteeringColumn_pivot_Fiat_Bravo_1) -> SteeringColumn_pivot_Fiat_Bravo_1/1(SteeringColumn_pivot_Fiat_Bravo_1)
  Fiat_Bravo_1/8(Fiat_Bravo_1_Brake_light_center) -> Fiat_Bravo_1_Brake_light_center/1(Fiat_Bravo_1_Brake_light_center)
  Fiat_Bravo_1/9(Fiat_Bravo_1_Brake_light_left) -> Fiat_Bravo_1_Brake_light_left/1(Fiat_Bravo_1_Brake_light_left)
  Fiat_Bravo_1/10(Fiat_Bravo_1_Brake_light_right) -> Fiat_Bravo_1_Brake_light_right/1(Fiat_Bravo_1_Brake_light_right)
  Fiat_Bravo_1/11(Fiat_Bravo_1_Indicator_front_left) -> Fiat_Bravo_1_Indicator_front_left/1(Fiat_Bravo_1_Indicator_front_left)
  Fiat_Bravo_1/12(Fiat_Bravo_1_Indicator_side_left) -> Fiat_Bravo_1_Indicator_side_left/1(Fiat_Bravo_1_Indicator_side_left)
  Fiat_Bravo_1/13(Fiat_Bravo_1_Indicator_rear_left) -> Fiat_Bravo_1_Indicator_rear_left/1(Fiat_Bravo_1_Indicator_rear_left)
  Fiat_Bravo_1/14(Fiat_Bravo_1_Indicator_front_right) -> Fiat_Bravo_1_Indicator_front_right/1(Fiat_Bravo_1_Indicator_front_right)
  Fiat_Bravo_1/15(Fiat_Bravo_1_Indicator_side_right) -> Fiat_Bravo_1_Indicator_side_right/1(Fiat_Bravo_1_Indicator_side_right)
  Fiat_Bravo_1/16(Fiat_Bravo_1_Indicator_rear_right) -> Fiat_Bravo_1_Indicator_rear_right/1(Fiat_Bravo_1_Indicator_rear_right)
  Actros_2541_2/1(STATE_Actros_2541_2_bus) -> STATE_Actros_2541_2_bus/1(STATE_Actros_2541_2_bus)
  SELF_Actros_2541_2/1(SELF_Actros_2541_2) -> Actros_2541_2/1(SELF_Actros_2541_2)
  Actros_2541_3/1(STATE_Actros_2541_3_bus) -> STATE_Actros_2541_3_bus/1(STATE_Actros_2541_3_bus)
  SELF_Actros_2541_3/1(SELF_Actros_2541_3) -> Actros_2541_3/1(SELF_Actros_2541_3)
  Actros_2541_3/2(SteeringWheel_pivot_Actros_2541_3) -> SteeringWheel_pivot_Actros_2541_3/1(SteeringWheel_pivot_Actros_2541_3)
  Actros_2541_3/3(SteeringColumn_pivot_Actros_2541_3) -> SteeringColumn_pivot_Actros_2541_3/1(SteeringColumn_pivot_Actros_2541_3)
  Actros_2541_3/4(Actros_2541_3_Brake_light_left) -> Actros_2541_3_Brake_light_left/1(Actros_2541_3_Brake_light_left)
  Actros_2541_3/5(Actros_2541_3_Brake_light_right) -> Actros_2541_3_Brake_light_right/1(Actros_2541_3_Brake_light_right)
  Actros_2541_3/6(Actros_2541_3_Indicator_front_left) -> Actros_2541_3_Indicator_front_left/1(Actros_2541_3_Indicator_front_left)
  Actros_2541_3/7(Actros_2541_3_Indicator_side_left_1) -> Actros_2541_3_Indicator_side_left_1/1(Actros_2541_3_Indicator_side_left_1)
  Actros_2541_3/8(Actros_2541_3_Indicator_side_left_2) -> Actros_2541_3_Indicator_side_left_2/1(Actros_2541_3_Indicator_side_left_2)
  Actros_2541_3/9(Actros_2541_3_Indicator_side_left_3) -> Actros_2541_3_Indicator_side_left_3/1(Actros_2541_3_Indicator_side_left_3)
  Actros_2541_3/10(Actros_2541_3_Indicator_rear_left) -> Actros_2541_3_Indicator_rear_left/1(Actros_2541_3_Indicator_rear_left)
  Actros_2541_3/11(Actros_2541_3_Indicator_front_right) -> Actros_2541_3_Indicator_front_right/1(Actros_2541_3_Indicator_front_right)
  Actros_2541_3/12(Actros_2541_3_Indicator_side_right_1) -> Actros_2541_3_Indicator_side_right_1/1(Actros_2541_3_Indicator_side_right_1)
  Actros_2541_3/13(Actros_2541_3_Indicator_side_right_2) -> Actros_2541_3_Indicator_side_right_2/1(Actros_2541_3_Indicator_side_right_2)
  Actros_2541_3/14(Actros_2541_3_Indicator_side_right_3) -> Actros_2541_3_Indicator_side_right_3/1(Actros_2541_3_Indicator_side_right_3)
  Actros_2541_3/15(Actros_2541_3_Indicator_rear_right) -> Actros_2541_3_Indicator_rear_right/1(Actros_2541_3_Indicator_rear_right)
  Mazda_RX8_1/1(STATE_Mazda_RX8_1_bus) -> STATE_Mazda_RX8_1_bus/1(STATE_Mazda_RX8_1_bus)
  SELF_Mazda_RX8_1/1(SELF_Mazda_RX8_1) -> Mazda_RX8_1/1(SELF_Mazda_RX8_1)
  Citroen_C3_2/1(STATE_Citroen_C3_2_bus) -> STATE_Citroen_C3_2_bus/1(STATE_Citroen_C3_2_bus)
  SELF_Citroen_C3_2/1(SELF_Citroen_C3_2) -> Citroen_C3_2/1(SELF_Citroen_C3_2)
  Toyota_Yaris_1/1(STATE_Toyota_Yaris_1_bus) -> STATE_Toyota_Yaris_1_bus/1(STATE_Toyota_Yaris_1_bus)
  SELF_Toyota_Yaris_1/1(SELF_Toyota_Yaris_1) -> Toyota_Yaris_1/1(SELF_Toyota_Yaris_1)
  Actros_2541_4/1(STATE_Actros_2541_4_bus) -> STATE_Actros_2541_4_bus/1(STATE_Actros_2541_4_bus)
  SELF_Actros_2541_4/1(SELF_Actros_2541_4) -> Actros_2541_4/1(SELF_Actros_2541_4)
  Daf_95_1/1(STATE_Daf_95_1_bus) -> STATE_Daf_95_1_bus/1(STATE_Daf_95_1_bus)
  SELF_Daf_95_1/1(SELF_Daf_95_1) -> Daf_95_1/1(SELF_Daf_95_1)
  Ford_Fiesta_1/1(STATE_Ford_Fiesta_1_bus) -> STATE_Ford_Fiesta_1_bus/1(STATE_Ford_Fiesta_1_bus)
  SELF_Ford_Fiesta_1/1(SELF_Ford_Fiesta_1) -> Ford_Fiesta_1/1(SELF_Ford_Fiesta_1)
  Honda_Pan_European_1/1(STATE_Honda_Pan_European_1_bus) -> STATE_Honda_Pan_European_1_bus/1(STATE_Honda_Pan_European_1_bus)
  SELF_Honda_Pan_European_1/1(SELF_Honda_Pan_European_1) -> Honda_Pan_European_1/1(SELF_Honda_Pan_European_1)
  Nissan_Cabstar_2/1(STATE_Nissan_Cabstar_2_bus) -> STATE_Nissan_Cabstar_2_bus/1(STATE_Nissan_Cabstar_2_bus)
  SELF_Nissan_Cabstar_2/1(SELF_Nissan_Cabstar_2) -> Nissan_Cabstar_2/1(SELF_Nissan_Cabstar_2)
  BMW_X5_1/1(STATE_BMW_X5_1_bus) -> STATE_BMW_X5_1_bus/1(STATE_BMW_X5_1_bus)
  SELF_BMW_X5_1/1(SELF_BMW_X5_1) -> BMW_X5_1/1(SELF_BMW_X5_1)
  Nissan_Cabstar_3/1(STATE_Nissan_Cabstar_3_bus) -> STATE_Nissan_Cabstar_3_bus/1(STATE_Nissan_Cabstar_3_bus)
  SELF_Nissan_Cabstar_3/1(SELF_Nissan_Cabstar_3) -> Nissan_Cabstar_3/1(SELF_Nissan_Cabstar_3)
  Male_RegularAni_1/1(STATE_Male_RegularAni_1_bus) -> STATE_Male_RegularAni_1_bus/1(STATE_Male_RegularAni_1_bus)
  Male_RegularAni_1/2(ANIM_Male_RegularAni_1) -> ANIM_Male_RegularAni_1/1(ANIM_Male_RegularAni_1)
  SELF_Male_RegularAni_1/1(SELF_Male_RegularAni_1) -> Male_RegularAni_1/1(SELF_Male_RegularAni_1)
  Male_RegularAni_1/3(VISUColorRegion_Upper_Body_Male_RegularAni_1) -> VISUColorRegion_Upper_Body_Male_RegularAni_1/1(VISUColorRegion_Upper_Body_Male_RegularAni_1)
  Male_RegularAni_1/4(VISUColorRegion_Lower_Body_Male_RegularAni_1) -> VISUColorRegion_Lower_Body_Male_RegularAni_1/1(VISUColorRegion_Lower_Body_Male_RegularAni_1)
  Male_RegularAni_1/5(VISUColorRegion_Shoes_Male_RegularAni_1) -> VISUColorRegion_Shoes_Male_RegularAni_1/1(VISUColorRegion_Shoes_Male_RegularAni_1)
  HighwayOverhang_1/1(VISUMatrixSign_HighwayOverhang_1) -> VISUMatrixSign_HighwayOverhang_1/1(VISUMatrixSign_HighwayOverhang_1)
  HighwayOverhang_1/2(VISUMatrixSignLights_HighwayOverhang_1) -> VISUMatrixSignLights_HighwayOverhang_1/1(VISUMatrixSignLights_HighwayOverhang_1)
  HighwayOverhang_2/1(VISUMatrixSign_HighwayOverhang_2) -> VISUMatrixSign_HighwayOverhang_2/1(VISUMatrixSign_HighwayOverhang_2)
  HighwayOverhang_2/2(VISUMatrixSignLights_HighwayOverhang_2) -> VISUMatrixSignLights_HighwayOverhang_2/1(VISUMatrixSignLights_HighwayOverhang_2)
  HighwayOverhang_3/1(VISUMatrixSign_HighwayOverhang_3) -> VISUMatrixSign_HighwayOverhang_3/1(VISUMatrixSign_HighwayOverhang_3)
  HighwayOverhang_3/2(VISUMatrixSignLights_HighwayOverhang_3) -> VISUMatrixSignLights_HighwayOverhang_3/1(VISUMatrixSignLights_HighwayOverhang_3)
  HighwayOverhang_4/1(VISUMatrixSign_HighwayOverhang_4) -> VISUMatrixSign_HighwayOverhang_4/1(VISUMatrixSign_HighwayOverhang_4)
  HighwayOverhang_4/2(VISUMatrixSignLights_HighwayOverhang_4) -> VISUMatrixSignLights_HighwayOverhang_4/1(VISUMatrixSignLights_HighwayOverhang_4)
  HighwayOverhang_5/1(VISUMatrixSign_HighwayOverhang_5) -> VISUMatrixSign_HighwayOverhang_5/1(VISUMatrixSign_HighwayOverhang_5)
  HighwayOverhang_5/2(VISUMatrixSignLights_HighwayOverhang_5) -> VISUMatrixSignLights_HighwayOverhang_5/1(VISUMatrixSignLights_HighwayOverhang_5)
  HighwayOverhang_6/1(VISUMatrixSign_HighwayOverhang_6) -> VISUMatrixSign_HighwayOverhang_6/1(VISUMatrixSign_HighwayOverhang_6)
  HighwayOverhang_6/2(VISUMatrixSignLights_HighwayOverhang_6) -> VISUMatrixSignLights_HighwayOverhang_6/1(VISUMatrixSignLights_HighwayOverhang_6)
  HighwayOverhang_7/1(VISUMatrixSign_HighwayOverhang_7) -> VISUMatrixSign_HighwayOverhang_7/1(VISUMatrixSign_HighwayOverhang_7)
  HighwayOverhang_7/2(VISUMatrixSignLights_HighwayOverhang_7) -> VISUMatrixSignLights_HighwayOverhang_7/1(VISUMatrixSignLights_HighwayOverhang_7)
  HighwayOverhang_8/1(VISUMatrixSign_HighwayOverhang_8) -> VISUMatrixSign_HighwayOverhang_8/1(VISUMatrixSign_HighwayOverhang_8)
  HighwayOverhang_8/2(VISUMatrixSignLights_HighwayOverhang_8) -> VISUMatrixSignLights_HighwayOverhang_8/1(VISUMatrixSignLights_HighwayOverhang_8)
  HighwayOverhang_9/1(VISUMatrixSign_HighwayOverhang_9) -> VISUMatrixSign_HighwayOverhang_9/1(VISUMatrixSign_HighwayOverhang_9)
  HighwayOverhang_9/2(VISUMatrixSignLights_HighwayOverhang_9) -> VISUMatrixSignLights_HighwayOverhang_9/1(VISUMatrixSignLights_HighwayOverhang_9)
  HighwayOverhang_10/1(VISUMatrixSign_HighwayOverhang_10) -> VISUMatrixSign_HighwayOverhang_10/1(VISUMatrixSign_HighwayOverhang_10)
  HighwayOverhang_10/2(VISUMatrixSignLights_HighwayOverhang_10) -> VISUMatrixSignLights_HighwayOverhang_10/1(VISUMatrixSignLights_HighwayOverhang_10)
  HighwayOverhang_11/1(VISUMatrixSign_HighwayOverhang_11) -> VISUMatrixSign_HighwayOverhang_11/1(VISUMatrixSign_HighwayOverhang_11)
  HighwayOverhang_11/2(VISUMatrixSignLights_HighwayOverhang_11) -> VISUMatrixSignLights_HighwayOverhang_11/1(VISUMatrixSignLights_HighwayOverhang_11)
  HighwayOverhang_12/1(VISUMatrixSign_HighwayOverhang_12) -> VISUMatrixSign_HighwayOverhang_12/1(VISUMatrixSign_HighwayOverhang_12)
  HighwayOverhang_12/2(VISUMatrixSignLights_HighwayOverhang_12) -> VISUMatrixSignLights_HighwayOverhang_12/1(VISUMatrixSignLights_HighwayOverhang_12)
  HighwayOverhang_13/1(VISUMatrixSign_HighwayOverhang_13) -> VISUMatrixSign_HighwayOverhang_13/1(VISUMatrixSign_HighwayOverhang_13)
  HighwayOverhang_13/2(VISUMatrixSignLights_HighwayOverhang_13) -> VISUMatrixSignLights_HighwayOverhang_13/1(VISUMatrixSignLights_HighwayOverhang_13)
  HighwayOverhang_14/1(VISUMatrixSign_HighwayOverhang_14) -> VISUMatrixSign_HighwayOverhang_14/1(VISUMatrixSign_HighwayOverhang_14)
  HighwayOverhang_14/2(VISUMatrixSignLights_HighwayOverhang_14) -> VISUMatrixSignLights_HighwayOverhang_14/1(VISUMatrixSignLights_HighwayOverhang_14)
  HighwayOverhang_15/1(VISUMatrixSign_HighwayOverhang_15) -> VISUMatrixSign_HighwayOverhang_15/1(VISUMatrixSign_HighwayOverhang_15)
  HighwayOverhang_15/2(VISUMatrixSignLights_HighwayOverhang_15) -> VISUMatrixSignLights_HighwayOverhang_15/1(VISUMatrixSignLights_HighwayOverhang_15)
  HighwayOverhang_16/1(VISUMatrixSign_HighwayOverhang_16) -> VISUMatrixSign_HighwayOverhang_16/1(VISUMatrixSign_HighwayOverhang_16)
  HighwayOverhang_16/2(VISUMatrixSignLights_HighwayOverhang_16) -> VISUMatrixSignLights_HighwayOverhang_16/1(VISUMatrixSignLights_HighwayOverhang_16)
  HighwayOverhang_17/1(VISUMatrixSign_HighwayOverhang_17) -> VISUMatrixSign_HighwayOverhang_17/1(VISUMatrixSign_HighwayOverhang_17)
  HighwayOverhang_17/2(VISUMatrixSignLights_HighwayOverhang_17) -> VISUMatrixSignLights_HighwayOverhang_17/1(VISUMatrixSignLights_HighwayOverhang_17)
  HighwayOverhang_18/1(VISUMatrixSign_HighwayOverhang_18) -> VISUMatrixSign_HighwayOverhang_18/1(VISUMatrixSign_HighwayOverhang_18)
  HighwayOverhang_18/2(VISUMatrixSignLights_HighwayOverhang_18) -> VISUMatrixSignLights_HighwayOverhang_18/1(VISUMatrixSignLights_HighwayOverhang_18)
  HighwayOverhang_20/1(VISUMatrixSign_HighwayOverhang_20) -> VISUMatrixSign_HighwayOverhang_20/1(VISUMatrixSign_HighwayOverhang_20)
  HighwayOverhang_20/2(VISUMatrixSignLights_HighwayOverhang_20) -> VISUMatrixSignLights_HighwayOverhang_20/1(VISUMatrixSignLights_HighwayOverhang_20)
  HighwayOverhang_19/1(VISUMatrixSign_HighwayOverhang_19) -> VISUMatrixSign_HighwayOverhang_19/1(VISUMatrixSign_HighwayOverhang_19)
  HighwayOverhang_19/2(VISUMatrixSignLights_HighwayOverhang_19) -> VISUMatrixSignLights_HighwayOverhang_19/1(VISUMatrixSignLights_HighwayOverhang_19)
  HighwayOverhang_21/1(VISUMatrixSign_HighwayOverhang_21) -> VISUMatrixSign_HighwayOverhang_21/1(VISUMatrixSign_HighwayOverhang_21)
  HighwayOverhang_21/2(VISUMatrixSignLights_HighwayOverhang_21) -> VISUMatrixSignLights_HighwayOverhang_21/1(VISUMatrixSignLights_HighwayOverhang_21)
  HighwayOverhang_22/1(VISUMatrixSign_HighwayOverhang_22) -> VISUMatrixSign_HighwayOverhang_22/1(VISUMatrixSign_HighwayOverhang_22)
  HighwayOverhang_22/2(VISUMatrixSignLights_HighwayOverhang_22) -> VISUMatrixSignLights_HighwayOverhang_22/1(VISUMatrixSignLights_HighwayOverhang_22)
  HighwayOverhang_23/1(VISUMatrixSign_HighwayOverhang_23) -> VISUMatrixSign_HighwayOverhang_23/1(VISUMatrixSign_HighwayOverhang_23)
  HighwayOverhang_23/2(VISUMatrixSignLights_HighwayOverhang_23) -> VISUMatrixSignLights_HighwayOverhang_23/1(VISUMatrixSignLights_HighwayOverhang_23)
  HighwayOverhang_24/1(VISUMatrixSign_HighwayOverhang_24) -> VISUMatrixSign_HighwayOverhang_24/1(VISUMatrixSign_HighwayOverhang_24)
  HighwayOverhang_24/2(VISUMatrixSignLights_HighwayOverhang_24) -> VISUMatrixSignLights_HighwayOverhang_24/1(VISUMatrixSignLights_HighwayOverhang_24)
  HighwayOverhang_25/1(VISUMatrixSign_HighwayOverhang_25) -> VISUMatrixSign_HighwayOverhang_25/1(VISUMatrixSign_HighwayOverhang_25)
  HighwayOverhang_25/2(VISUMatrixSignLights_HighwayOverhang_25) -> VISUMatrixSignLights_HighwayOverhang_25/1(VISUMatrixSignLights_HighwayOverhang_25)
  HighwayOverhang_26/1(VISUMatrixSign_HighwayOverhang_26) -> VISUMatrixSign_HighwayOverhang_26/1(VISUMatrixSign_HighwayOverhang_26)
  HighwayOverhang_26/2(VISUMatrixSignLights_HighwayOverhang_26) -> VISUMatrixSignLights_HighwayOverhang_26/1(VISUMatrixSignLights_HighwayOverhang_26)
  HighwayOverhang_27/1(VISUMatrixSign_HighwayOverhang_27) -> VISUMatrixSign_HighwayOverhang_27/1(VISUMatrixSign_HighwayOverhang_27)
  HighwayOverhang_27/2(VISUMatrixSignLights_HighwayOverhang_27) -> VISUMatrixSignLights_HighwayOverhang_27/1(VISUMatrixSignLights_HighwayOverhang_27)
  HighwayOverhang_28/1(VISUMatrixSign_HighwayOverhang_28) -> VISUMatrixSign_HighwayOverhang_28/1(VISUMatrixSign_HighwayOverhang_28)
  HighwayOverhang_28/2(VISUMatrixSignLights_HighwayOverhang_28) -> VISUMatrixSignLights_HighwayOverhang_28/1(VISUMatrixSignLights_HighwayOverhang_28)
